simulink model "queue_populator_modeling"  (R2020b)
settings: Solver=FixedStepDiscrete  StartTime=0.0  StopTime=10.0  FixedStep=0.1  RelTol=1e-3
undefined symbols (not defined in the file): container_values, first_index, last_queue_index
settings Model: Creator=rsub  LastModifiedBy=rsub

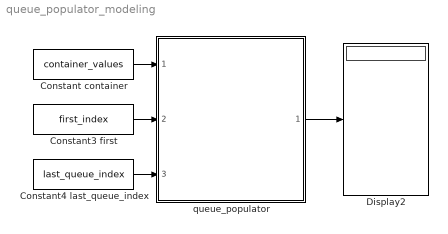
== system queue_populator_modeling ==
  Constant container : Constant  Value=container_values
  Constant3 first : Constant  Value=first_index
  Constant4 last_queue_index : Constant  Value=last_queue_index
  Display2 : Display
  queue_populator : Subsystem  ReferencedSubsystem=queue_populator_model
  wires:
  queue_populator/1 -> Display2/1
  Constant4 last_queue_index/1 -> queue_populator/3
  Constant3 first/1 -> queue_populator/2
  Constant container/1 -> queue_populator/1
